simulink library "INT_EngReq_TrqLimCalc"  (R2016b)
settings: Solver=VariableStepAuto  StartTime=0.0  StopTime=10.0  RelTol=1e-3
settings Model: Creator=Administrator  LastModifiedBy=Administrator

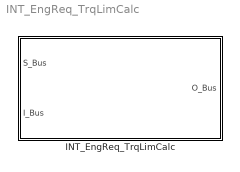
== system INT_EngReq_TrqLimCalc ==
  INT_EngReq_TrqLimCalc : Subsystem

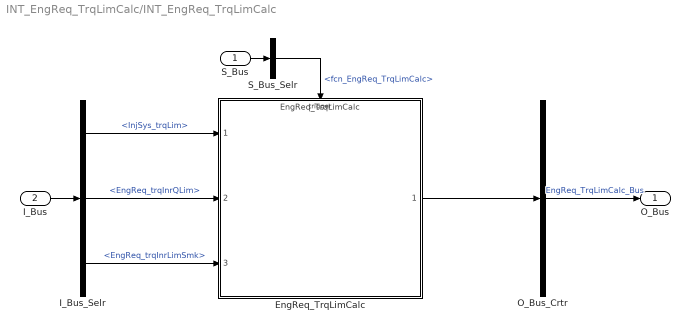
== system INT_EngReq_TrqLimCalc/INT_EngReq_TrqLimCalc ==
  S_Bus : Inport
  I_Bus : Inport  Port=2
  EngReq_TrqLimCalc : ModelReference  ModelNameDialog=EngReq_TrqLimCalc  SimulationMode=Normal  ModelReferenceVersion=1.11  TriggerPortName=function  TriggerPortTriggerType=function-call  TriggerPortStatesWhenEnabling=held
  I_Bus_Selr : BusSelector  OutputSignals=InjSys_trqLim,EngReq_trqInrQLim,EngReq_trqInrLimSmk
  O_Bus_Crtr : BusCreator  Inputs=1
  S_Bus_Selr : BusSelector  OutputSignals=fcn_EngReq_TrqLimCalc
  O_Bus : Outport
  wires:
  S_Bus_Selr/1 -> EngReq_TrqLimCalc/Trigger  "<fcn_EngReq_TrqLimCalc>"
  S_Bus/1 -> S_Bus_Selr/1
  I_Bus/1 -> I_Bus_Selr/1
  I_Bus_Selr/1 -> EngReq_TrqLimCalc/1  "<InjSys_trqLim>"
  I_Bus_Selr/2 -> EngReq_TrqLimCalc/2  "<EngReq_trqInrQLim>"
  I_Bus_Selr/3 -> EngReq_TrqLimCalc/3  "<EngReq_trqInrLimSmk>"
  O_Bus_Crtr/1 -> O_Bus/1  "EngReq_TrqLimCalc_Bus"
  EngReq_TrqLimCalc/1 -> O_Bus_Crtr/1
